simulink model "Node_M"  (R2024b)
settings: Solver=ode1  StartTime=0.0  StopTime=10.0  FixedStep=0.5e-3  RelTol=1e-3
libraries: simulink x1
settings Model: DataDictionary=M_dd.sldd  EnableAccessToBaseWorkspace=off  Creator=wai484  LastModifiedBy=wai484
settings SolverCC: EnableFixedStepZeroCrossing=on
settings DataIOCC: SaveOutput=off  SignalLogging=off  DSMLogging=off  SaveTime=off  ReturnWorkspaceOutputs=off
settings OptimizationCC: UseDivisionForNetSlopeComputation=UseDivisionForReciprocalsOfIntegersOnly  StateBitsets=on  DataBitsets=on  EfficientMapNaN2IntZero=off  SimCompilerOptimization=on
settings DebuggingCC: SignalInfNanChecking=error  SignalRangeChecking=error  ReadBeforeWriteMsg=EnableAllAsError  WriteAfterWriteMsg=EnableAllAsError  WriteAfterReadMsg=EnableAllAsError  AlgebraicLoopMsg=error  ArtificialAlgebraicLoopMsg=error  SaveWithDisabledLinksMsg=error  SaveWithParameterizedLinksMsg=error  BlockPriorityViolationMsg=error  SolverPrmCheckMsg=error  InheritedTsInSrcMsg=error  TasksWithSamePriorityMsg=error  SigSpecEnsureSampleTimeMsg=error  CheckMatrixSingularityMsg=error  IntegerOverflowMsg=error  ParameterUnderflowMsg=error  ParameterPrecisionLossMsg=error  ParameterTunabilityLossMsg=error  UnderSpecifiedDataTypeMsg=error  UnnecessaryDatatypeConvMsg=warning  VectorMatrixConversionMsg=error  UnconnectedInputMsg=error  UnconnectedOutputMsg=error  UnconnectedLineMsg=error  SFcnCompatibilityMsg=error  UniqueDataStoreMsg=error  BusObjectLabelMismatch=error  RootOutportRequireBusObject=error  AssertControl=DisableAll  ModelReferenceIOMismatchMessage=error  UnknownTsInhSupMsg=error  ModelReferenceDataLoggingMessage=error  StateNameClashWarn=warning  StrictBusMsg=ErrorOnBusTreatedAsVector  NonBusSignalsTreatedAsBus=error  SFUnusedDataAndEventsDiag=error  SFInvalidInputDataAccessInChartInitDiag=error  SFTransitionOutsideNaturalParentDiag=error  SFUnreachableExecutionPathDiag=error  SFUndirectedBroadcastEventsDiag=error  SFTransitionActionBeforeConditionDiag=error  SFTemporalDelaySmallerThanSampleTimeDiag=error  SFSelfTransitionDiag=error  SFExecutionAtInitializationDiag=error  IntegerSaturationMsg=error  VariantConditionMismatch=error
settings ModelReferenceCC: EnableParallelModelReferenceBuilds=on
settings SFSimCC: CompileTimeRecursionLimit=0  EnableRuntimeRecursion=off  MATLABDynamicMemAlloc=off  SimHardwareAcceleration=native
settings RTWCC: BuildConfiguration=Faster Runs
settings GRTTargetCC: UtilityFuncGeneration=Shared location  MatFileLogging=off  SupportNonFinite=off  OptimizeReductions=on

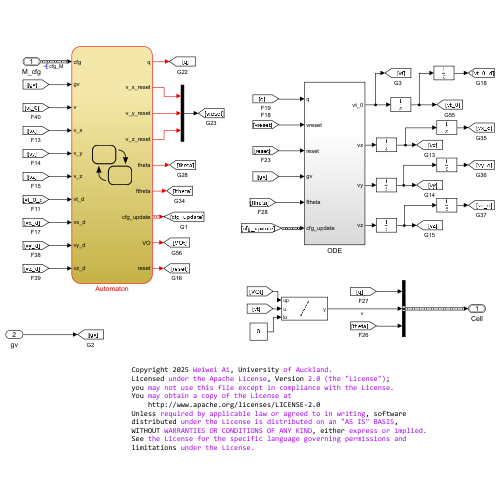
[thumbnail: Simulink's stored preview of the top-level diagram]
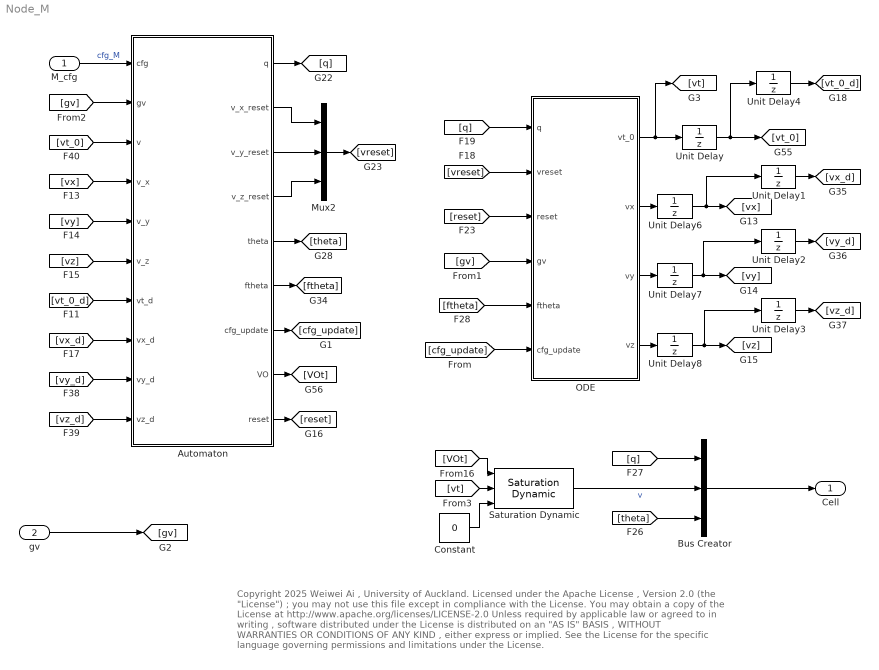
== system Node_M ==
  note: Copyright 2025 Weiwei Ai , University of Auckland.
      | Licensed under the Apache License , Version 2.0 (the "License") ;
      | you may not use this file except in compliance with the License.
      | You may obtain a copy of the License at
      | http://www.apache.org/licenses/LICENSE-2.0
      | Unless required by applicable law or agreed to in writing , software
      | distributed under the License is distributed on an "AS IS" BASIS ,
      | WITHOUT WARRANTIES OR CONDITIONS OF ANY KIND , either express or implied.
      | See the License for the specific language governing permissions and
      | limitations under the License.
  M_cfg : Inport  OutDataTypeStr=Bus: Config_M  BusOutputAsStruct=on
  gv : Inport  Port=2  OutDataTypeStr=double  PortDimensions=1
  Automaton : Stateflow chart  TreatAsAtomicUnit=on
  Bus Creator : BusCreator  Inputs=3  OutDataTypeStr=Bus: Cell  NonVirtualBus=on
      settings: InheritFromInputs=off
  Constant : Constant  Value=0
  Mux2 : Mux  Inputs=3
  ODE : Subsystem
  Saturation Dynamic : simulink/Discontinuities/Saturation Dynamic  OutMin=[]  OutMax=[]  OutDataTypeStr=Inherit: Same as second input  OutDataType=fixdt(1, 16)  OutScaling=2^-10  DoSatur=off
  Unit Delay{,1..4,6..8} (8 alike) : UnitDelay  SampleTime=-1  HasFrameUpgradeWarning=on
  Cell : Outport  OutDataTypeStr=Bus: Cell
  wires:
  Automaton/2(v_x_reset) -> Mux2/1
  Automaton/3(v_y_reset) -> Mux2/2
  Automaton/4(v_z_reset) -> Mux2/3
  Automaton/9(reset) -> [reset]
  Mux2/1 -> [vreset]
  Automaton/1(q) -> [q]
  [q] -> ODE/1(q)
  [q] -> Bus Creator/1
  [theta] -> Bus Creator/3
  [ftheta] -> ODE/5(ftheta)
  Automaton/5(theta) -> [theta]
  ODE/1(vt_0) -> [vt], Unit Delay/1
  Unit Delay/1 -> Unit Delay4/1, [vt_0]
  [vt] -> Saturation Dynamic/2
  [VOt] -> Saturation Dynamic/1
  Constant/1 -> Saturation Dynamic/3
  Saturation Dynamic/1 -> Bus Creator/2  "v"
  M_cfg/1 -> Automaton/1(cfg)  "cfg_M"
  [vt_0_d] -> Automaton/7(vt_d)
  [vt_0] -> Automaton/3(v)
  [vx] -> Automaton/4(v_x)
  [vz_d] -> Automaton/10(vz_d)
  [vy_d] -> Automaton/9(vy_d)
  [vx_d] -> Automaton/8(vx_d)
  [vz] -> Automaton/6(v_z)
  [vy] -> Automaton/5(v_y)
  Automaton/8(VO) -> [VOt]
  Automaton/6(ftheta) -> [ftheta]
  Automaton/7(cfg_update) -> [cfg_update]
  [reset] -> ODE/3(reset)
  [vreset] -> ODE/2(vreset)
  [gv] -> ODE/4(gv)
  [gv] -> Automaton/2(gv)
  ODE/4(vz) -> Unit Delay8/1
  Unit Delay1/1 -> [vx_d]
  Unit Delay2/1 -> [vy_d]
  Unit Delay3/1 -> [vz_d]
  [cfg_update] -> ODE/6(cfg_update)
  ODE/2(vx) -> Unit Delay6/1
  Unit Delay6/1 -> Unit Delay1/1, [vx]
  Unit Delay7/1 -> Unit Delay2/1, [vy]
  Unit Delay8/1 -> Unit Delay3/1, [vz]
  ODE/3(vy) -> Unit Delay7/1
  Unit Delay4/1 -> [vt_0_d]
  gv/1 -> [gv]
  Bus Creator/1 -> Cell/1

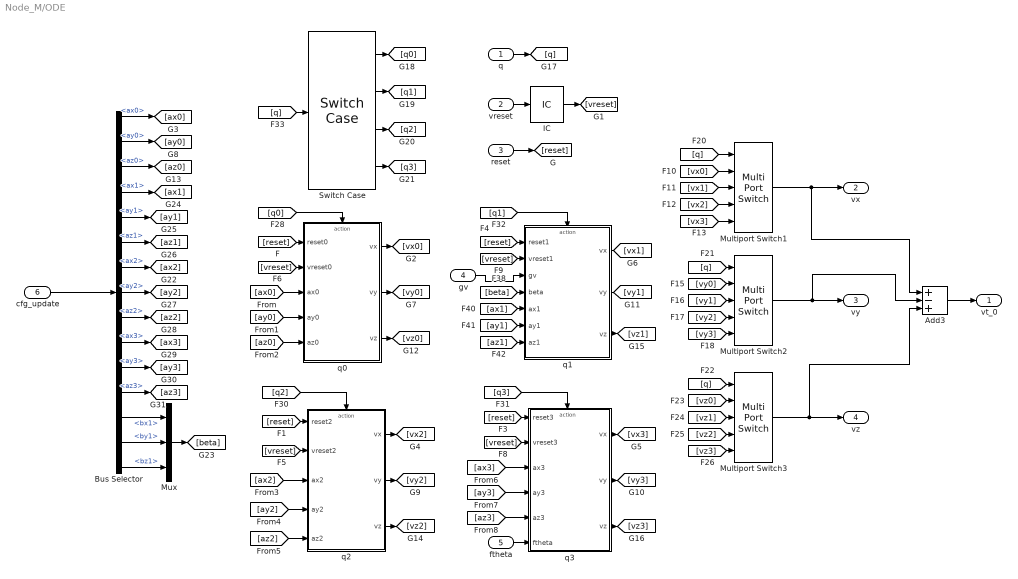
== system Node_M/ODE ==
  q : Inport
  vreset : Inport  Port=2
  reset : Inport  Port=3
  gv : Inport  Port=4
  ftheta : Inport  Port=5
  cfg_update : Inport  Port=6  OutDataTypeStr=Bus: Config_M
  Add3 : Sum  Inputs=+-+
  Bus Selector : BusSelector  OutputSignals=ax0,ay0,az0,ax1,ay1,az1,ax2,ay2,az2,ax3,ay3,az3,bx1,by1,bz1
  IC : InitialCondition  Value=0
  Multiport Switch1 : MultiPortSwitch  DataPortOrder=Zero-based contiguous  Inputs=4  zeroidx=on  SaturateOnIntegerOverflow=off  InputSameDT=off
  Multiport Switch2 : MultiPortSwitch  DataPortOrder=Zero-based contiguous  Inputs=4  zeroidx=on  SaturateOnIntegerOverflow=off  InputSameDT=off
  Multiport Switch3 : MultiPortSwitch  DataPortOrder=Zero-based contiguous  Inputs=4  zeroidx=on  SaturateOnIntegerOverflow=off  InputSameDT=off
  Mux : Mux  Inputs=3
  Switch Case : SwitchCase  CaseConditions={0,1,2,3}  ShowDefaultCase=off
  q0 : Subsystem  TreatAsAtomicUnit=on
  q1 : Subsystem  TreatAsAtomicUnit=on
  q2 : Subsystem  TreatAsAtomicUnit=on
  q3 : Subsystem  TreatAsAtomicUnit=on
  vt_0 : Outport
  vx : Outport  Port=2
  vy : Outport  Port=3
  vz : Outport  Port=4
  wires:
  [az3] -> q3/5(az3)
  [az1] -> q1/7(az1)
  [ay1] -> q1/6(ay1)
  [ax1] -> q1/5(ax1)
  [beta] -> q1/4(beta)
  Mux/1 -> [beta]
  [q] -> Switch Case/1
  [q1] -> q1/Action
  [q3] -> q3/Action
  [q2] -> q2/Action
  [q0] -> q0/Action
  Switch Case/4 -> [q3]
  Switch Case/3 -> [q2]
  Switch Case/2 -> [q1]
  Switch Case/1 -> [q0]
  Multiport Switch3/1 -> vz/1, Add3/3
  [vz3] -> Multiport Switch3/5
  [vz2] -> Multiport Switch3/4
  [vz1] -> Multiport Switch3/3
  [vz0] -> Multiport Switch3/2
  [q] -> Multiport Switch3/1
  [q] -> Multiport Switch2/1
  [q] -> Multiport Switch1/1
  [vy3] -> Multiport Switch2/5
  [vy2] -> Multiport Switch2/4
  [vy1] -> Multiport Switch2/3
  [vy0] -> Multiport Switch2/2
  [vx3] -> Multiport Switch1/5
  [vx2] -> Multiport Switch1/4
  [vx1] -> Multiport Switch1/3
  [vx0] -> Multiport Switch1/2
  q1/3(vz) -> [vz1]
  q1/2(vy) -> [vy1]
  q1/1(vx) -> [vx1]
  q3/3(vz) -> [vz3]
  q3/2(vy) -> [vy3]
  q3/1(vx) -> [vx3]
  q2/2(vy) -> [vy2]
  q2/1(vx) -> [vx2]
  q2/3(vz) -> [vz2]
  q0/3(vz) -> [vz0]
  q0/2(vy) -> [vy0]
  q0/1(vx) -> [vx0]
  [vreset] -> q1/2(vreset1)
  [vreset] -> q3/2(vreset3)
  [vreset] -> q0/2(vreset0)
  [vreset] -> q2/2(vreset2)
  [reset] -> q1/1(reset1)
  [reset] -> q3/1(reset3)
  [reset] -> q2/1(reset2)
  [reset] -> q0/1(reset0)
  ftheta/1 -> q3/6(ftheta)
  [ax3] -> q3/3(ax3)
  Add3/1 -> vt_0/1
  [ax2] -> q2/3(ax2)
  q/1 -> [q]
  [ax0] -> q0/3(ax0)
  reset/1 -> [reset]
  [ay0] -> q0/4(ay0)
  [az0] -> q0/5(az0)
  [ay2] -> q2/4(ay2)
  [az2] -> q2/5(az2)
  [ay3] -> q3/4(ay3)
  vreset/1 -> IC/1
  IC/1 -> [vreset]
  Multiport Switch1/1 -> vx/1, Add3/1
  Multiport Switch2/1 -> vy/1, Add3/2
  gv/1 -> q1/3(gv)
  Bus Selector/4 -> [ax1]  "<ax1>"
  Bus Selector/5 -> [ay1]  "<ay1>"
  Bus Selector/6 -> [az1]  "<az1>"
  Bus Selector/1 -> [ax0]  "<ax0>"
  Bus Selector/2 -> [ay0]  "<ay0>"
  Bus Selector/3 -> [az0]  "<az0>"
  Bus Selector/7 -> [ax2]  "<ax2>"
  Bus Selector/8 -> [ay2]  "<ay2>"
  Bus Selector/9 -> [az2]  "<az2>"
  Bus Selector/10 -> [ax3]  "<ax3>"
  Bus Selector/11 -> [ay3]  "<ay3>"
  Bus Selector/12 -> [az3]  "<az3>"
  Bus Selector/13 -> Mux/1  "<bx1>"
  Bus Selector/14 -> Mux/2  "<by1>"
  Bus Selector/15 -> Mux/3  "<bz1>"
  cfg_update/1 -> Bus Selector/1

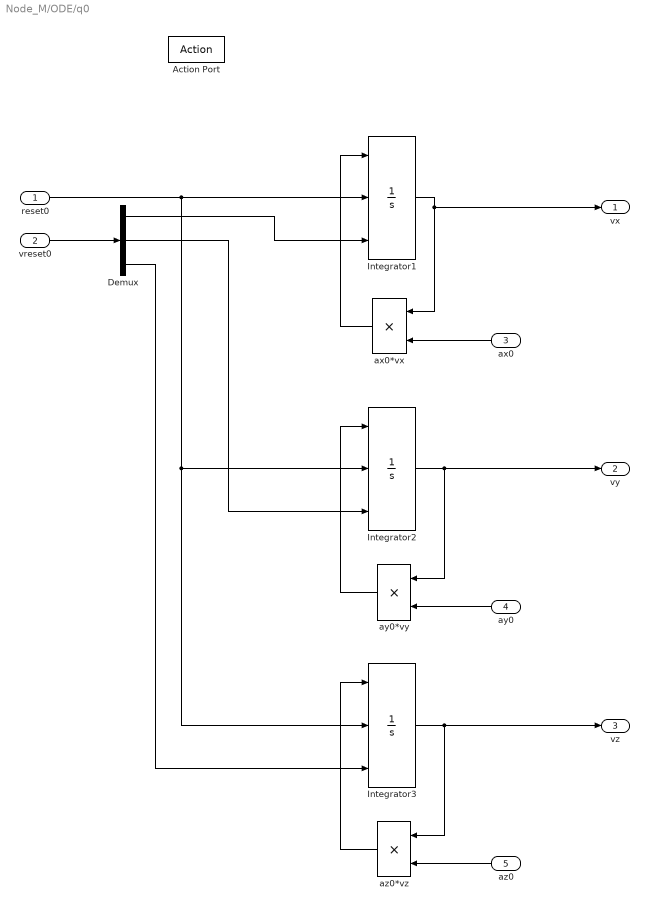
== system Node_M/ODE/q0 ==
  reset0 : Inport
  vreset0 : Inport  Port=2
  ax0 : Inport  Port=3
  ay0 : Inport  Port=4
  az0 : Inport  Port=5
  Action Port : ActionPort  InitializeStates=reset  ActionPortLabel=case [ 0 ]:
  Demux : Demux  Outputs=3
  Integrator1 : Integrator  ExternalReset=either  InitialConditionSource=external  InitialCondition=20
  Integrator2 : Integrator  ExternalReset=either  InitialConditionSource=external  InitialCondition=20
  Integrator3 : Integrator  ExternalReset=either  InitialConditionSource=external  InitialCondition=20
  ax0*vx : Product
  ay0*vy : Product
  az0*vz : Product
  vx : Outport
  vy : Outport  Port=2
  vz : Outport  Port=3
  wires:
  reset0/1 -> Integrator3/2, Integrator2/2, Integrator1/2
  ax0*vx/1 -> Integrator1/1
  Integrator1/1 -> ax0*vx/1, vx/1
  Integrator2/1 -> ay0*vy/1, vy/1
  ay0*vy/1 -> Integrator2/1
  Integrator3/1 -> vz/1, az0*vz/1
  az0*vz/1 -> Integrator3/1
  vreset0/1 -> Demux/1
  Demux/1 -> Integrator1/3
  Demux/2 -> Integrator2/3
  Demux/3 -> Integrator3/3
  ax0/1 -> ax0*vx/2
  ay0/1 -> ay0*vy/2
  az0/1 -> az0*vz/2

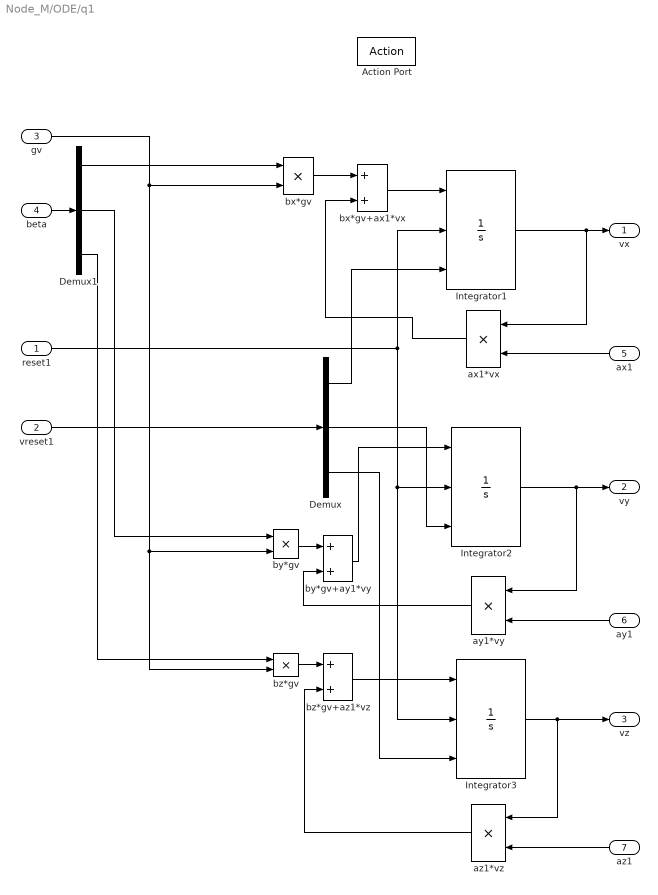
== system Node_M/ODE/q1 ==
  reset1 : Inport
  vreset1 : Inport  Port=2
  gv : Inport  Port=3
  beta : Inport  Port=4
  ax1 : Inport  Port=5
  ay1 : Inport  Port=6
  az1 : Inport  Port=7
  Action Port : ActionPort  InitializeStates=reset  ActionPortLabel=case [ 1 ]:
  Demux : Demux  Outputs=3
  Demux1 : Demux  Outputs=3
  Integrator1 : Integrator  ExternalReset=either  InitialConditionSource=external  InitialCondition=1
  Integrator2 : Integrator  ExternalReset=either  InitialConditionSource=external  InitialCondition=1
  Integrator3 : Integrator  ExternalReset=either  InitialConditionSource=external  InitialCondition=1
  ax1*vx : Product
  ay1*vy : Product
  az1*vz : Product
  bx*gv : Product
  bx*gv+ax1*vx : Sum
  by*gv : Product
  by*gv+ay1*vy : Sum
  bz*gv : Product
  bz*gv+az1*vz : Sum
  vx : Outport
  vy : Outport  Port=2
  vz : Outport  Port=3
  wires:
  Demux1/3 -> bz*gv/1
  Demux1/1 -> bx*gv/1
  beta/1 -> Demux1/1
  vreset1/1 -> Demux/1
  Integrator3/1 -> az1*vz/1, vz/1
  Integrator2/1 -> ay1*vy/1, vy/1
  Integrator1/1 -> vx/1, ax1*vx/1
  gv/1 -> bx*gv/2, by*gv/2, bz*gv/2
  reset1/1 -> Integrator1/2, Integrator2/2, Integrator3/2
  Demux/1 -> Integrator1/3
  Demux/2 -> Integrator2/3
  Demux/3 -> Integrator3/3
  az1/1 -> az1*vz/2
  bz*gv/1 -> bz*gv+az1*vz/1
  az1*vz/1 -> bz*gv+az1*vz/2
  bz*gv+az1*vz/1 -> Integrator3/1
  ay1/1 -> ay1*vy/2
  ay1*vy/1 -> by*gv+ay1*vy/2
  by*gv/1 -> by*gv+ay1*vy/1
  by*gv+ay1*vy/1 -> Integrator2/1
  bx*gv+ax1*vx/1 -> Integrator1/1
  ax1/1 -> ax1*vx/2
  bx*gv/1 -> bx*gv+ax1*vx/1
  ax1*vx/1 -> bx*gv+ax1*vx/2
  Demux1/2 -> by*gv/1

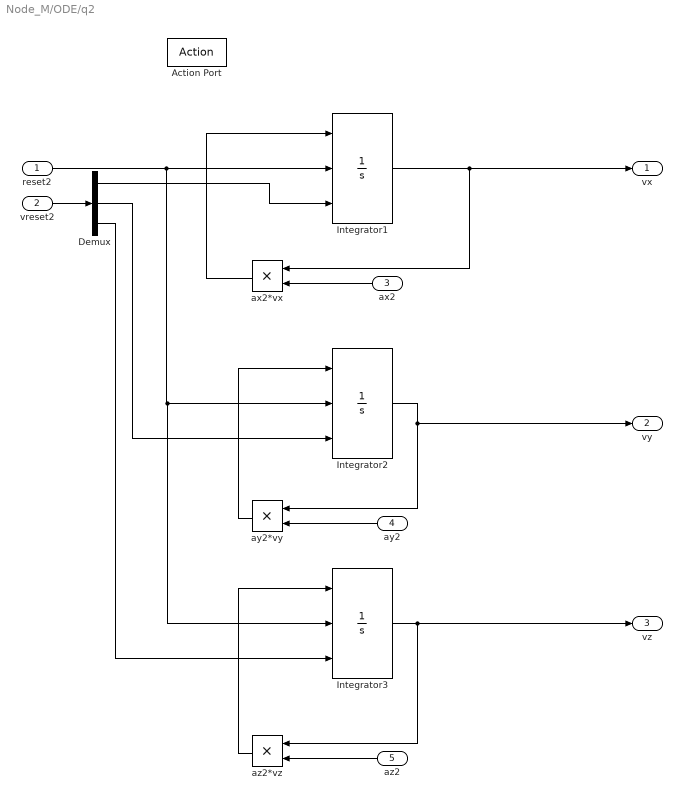
== system Node_M/ODE/q2 ==
  reset2 : Inport
  vreset2 : Inport  Port=2
  ax2 : Inport  Port=3
  ay2 : Inport  Port=4
  az2 : Inport  Port=5
  Action Port : ActionPort  InitializeStates=reset  ActionPortLabel=case [ 2 ]:
  Demux : Demux  Outputs=3
  Integrator1 : Integrator  ExternalReset=either  InitialConditionSource=external  InitialCondition=20
  Integrator2 : Integrator  ExternalReset=either  InitialConditionSource=external  InitialCondition=20
  Integrator3 : Integrator  ExternalReset=either  InitialConditionSource=external  InitialCondition=20
  ax2*vx : Product
  ay2*vy : Product
  az2*vz : Product
  vx : Outport
  vy : Outport  Port=2
  vz : Outport  Port=3
  wires:
  reset2/1 -> Integrator3/2, Integrator2/2, Integrator1/2
  ax2*vx/1 -> Integrator1/1
  ax2/1 -> ax2*vx/2
  Integrator1/1 -> ax2*vx/1, vx/1
  Integrator2/1 -> ay2*vy/1, vy/1
  ay2/1 -> ay2*vy/2
  Integrator3/1 -> az2*vz/1, vz/1
  az2/1 -> az2*vz/2
  ay2*vy/1 -> Integrator2/1
  az2*vz/1 -> Integrator3/1
  vreset2/1 -> Demux/1
  Demux/1 -> Integrator1/3
  Demux/2 -> Integrator2/3
  Demux/3 -> Integrator3/3

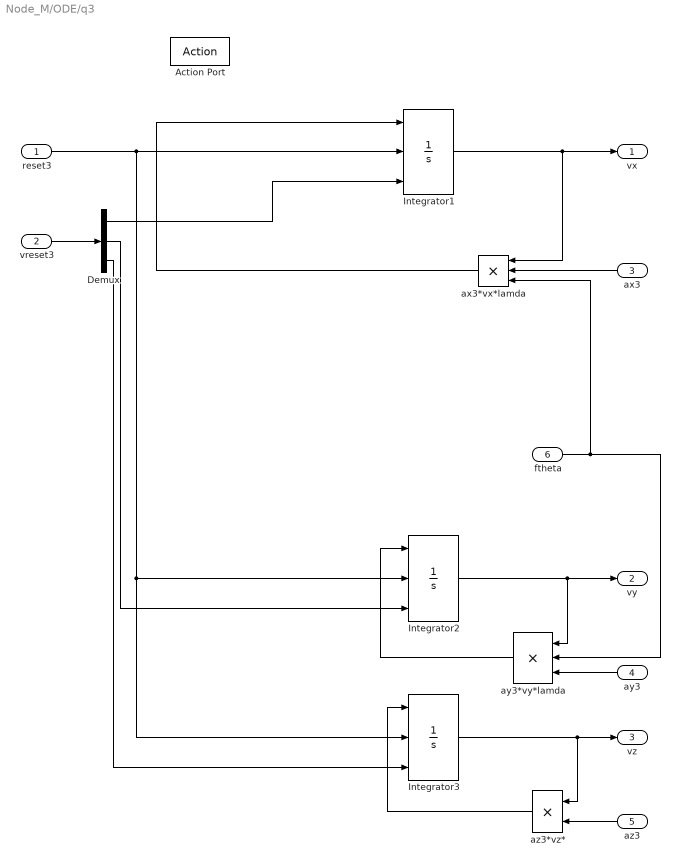
== system Node_M/ODE/q3 ==
  reset3 : Inport
  vreset3 : Inport  Port=2
  ax3 : Inport  Port=3
  ay3 : Inport  Port=4
  az3 : Inport  Port=5
  ftheta : Inport  Port=6
  Action Port : ActionPort  InitializeStates=reset  ActionPortLabel=case [ 3 ]:
  Demux : Demux  Outputs=3
  Integrator1 : Integrator  ExternalReset=either  InitialConditionSource=external  InitialCondition=133
  Integrator2 : Integrator  ExternalReset=either  InitialConditionSource=external  InitialCondition=133
  Integrator3 : Integrator  ExternalReset=either  InitialConditionSource=external  InitialCondition=133
  ax3*vx*lamda : Product  Inputs=3
  ay3*vy*lamda : Product  Inputs=3
  az3*vz* : Product
  vx : Outport
  vy : Outport  Port=2
  vz : Outport  Port=3
  wires:
  ftheta/1 -> ax3*vx*lamda/3, ay3*vy*lamda/2
  reset3/1 -> Integrator3/2, Integrator2/2, Integrator1/2
  ax3*vx*lamda/1 -> Integrator1/1
  ax3/1 -> ax3*vx*lamda/2
  Integrator1/1 -> ax3*vx*lamda/1, vx/1
  ay3*vy*lamda/1 -> Integrator2/1
  Integrator2/1 -> ay3*vy*lamda/1, vy/1
  Integrator3/1 -> az3*vz*/1, vz/1
  ay3/1 -> ay3*vy*lamda/3
  az3/1 -> az3*vz*/2
  az3*vz*/1 -> Integrator3/1
  vreset3/1 -> Demux/1
  Demux/1 -> Integrator1/3
  Demux/2 -> Integrator2/3
  Demux/3 -> Integrator3/3

== stateflow chart Node_M/Automaton ==
  state Resting_FR
    en: q=0;
    VT=cfg_update.VT;
  state Stimulated
    en: q=1;
  state Plateau_ER
    en:q=3;
  state Upstroke
    en: q=2;
  (default) -> Resting_FR : {cfg_update=cfg_default_M;}
  Resting_FR -> Stimulated : [(gv>VT)&&v<=VT]{...
      | VO_max=cfg_update.VO;
      | VR=cfg_update.VR;
      | v_x_reset=v_x;
      | v_y_reset=v_y;
      | v_z_reset=v_z;
      | vno=v;VO=VO_max-80.1*sqrt(vno/VR);
      | [theta,ftheta]=vtheta(vno,VR,cfg_update.a,cfg_update.b,cfg_update.c,cfg_update.d,cfg_update.e);
      | reset;}
  Stimulated -> Resting_FR [order 2] : [(gv<=0)&&v<VT]{...
      | v_x_reset=v_x;
      | v_y_reset=v_y;
      | v_z_reset=v_z;
      | reset;}
  Stimulated -> Upstroke [order 1] : [v>=VT]{...
      | v_x_reset=(v_x-vx_d)*(VT-vt_d)/(v-vt_d)+vx_d;
      | v_y_reset=(v_y-vy_d)*(VT-vt_d)/(v-vt_d)+vy_d;
      | v_z_reset=(v_z-vz_d)*(VT-vt_d)/(v-vt_d)+vz_d;
      | reset;}
  Plateau_ER -> Resting_FR : [v<=VR]{...
      | v_x_reset=(v_x-vx_d)*(VR-vt_d)/(v-vt_d)+vx_d;
      | v_y_reset=(v_y-vy_d)*(VR-vt_d)/(v-vt_d)+vy_d;
      | v_z_reset=(v_z-vz_d)*(VR-vt_d)/(v-vt_d)+vz_d;
      | cfg_update=cfg;
      | reset;}
  Upstroke -> Plateau_ER : [v>=VO]{...
      | v_x_reset=(v_x-vx_d)*(VO-vt_d)/(v-vt_d)+vx_d;
      | v_y_reset=(v_y-vy_d)*(VO-vt_d)/(v-vt_d)+vy_d;
      | v_z_reset=(v_z-vz_d)*(VO-vt_d)/(v-vt_d)+vz_d;
      | reset;}
  data: vnin function_input double; VRi function_input double; ain function_input double; bin function_input double; cin function_input double; din function_input double; ein function_input double; thetaout function_output double; fthetatout function_output double; cfg input Bus: Config_M; gv input; v input double; q output int8; v_x input; v_y input; v_z input; v_x_reset output double =0; v_y_reset output double =0; v_z_reset output double =0; vno local double; theta output double; ftheta output double; vt_d input double; vx_d input double; vy_d input double; vz_d input double; VO_max local; VR local; VT local; cfg_update output Bus: Config_M; VO output; cfg_default_M parameter Bus: Config_M
  events: reset output EITHER_EDGE_EVENT
  function [thetaout,fthetatout]  = vtheta(vnin,VRi,ain,bin,cin,din,ein):
    | function [thetaout,fthetatout]  = vtheta(vnin,VRi,ain,bin,cin,din,ein)
    | %Rate dependent factor
    | thetaout=vnin/VRi;
    | if thetaout<ein
    |     fthetatout=ain*exp(bin*thetaout)+cin*exp(-din*thetaout);
    | else
    |     fthetatout=ain*exp(bin*ein)+cin*exp(-din*ein);
    |     thetaout=ein;
    | end
    | 
    | end
